simulink model "ControlFuzzy_Modelo_GA"  (R2021b)
settings: Solver=VariableStepAuto  StartTime=0.0  StopTime=300  RelTol=1e-3
values from neighbouring files (symbols this model uses):
  Kd = 0.157560742107    [optimization_Result.mat]
  Ki = 0.0257835185528    [optimization_Result.mat]
  Kp = 1.9788581039    [optimization_Result.mat]
  Ku = 1.99972376218    [optimization_Result.mat]
libraries: fuzblock x1
settings Model: Creator=diego  LastModifiedBy=diego
settings SolverCC: ZeroCrossAlgorithm=Adaptive  AlgebraicLoopSolver=TrustRegion
settings DataIOCC: SaveOutput=off  SaveTime=off  ReturnWorkspaceOutputs=off
settings DebuggingCC: IgnoredZcDiagnostic=none  SFMachineParentedDataDiag=warning

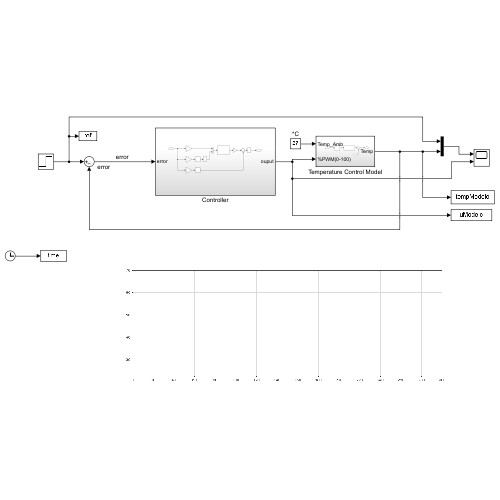
[thumbnail: Simulink's stored preview of the top-level diagram]
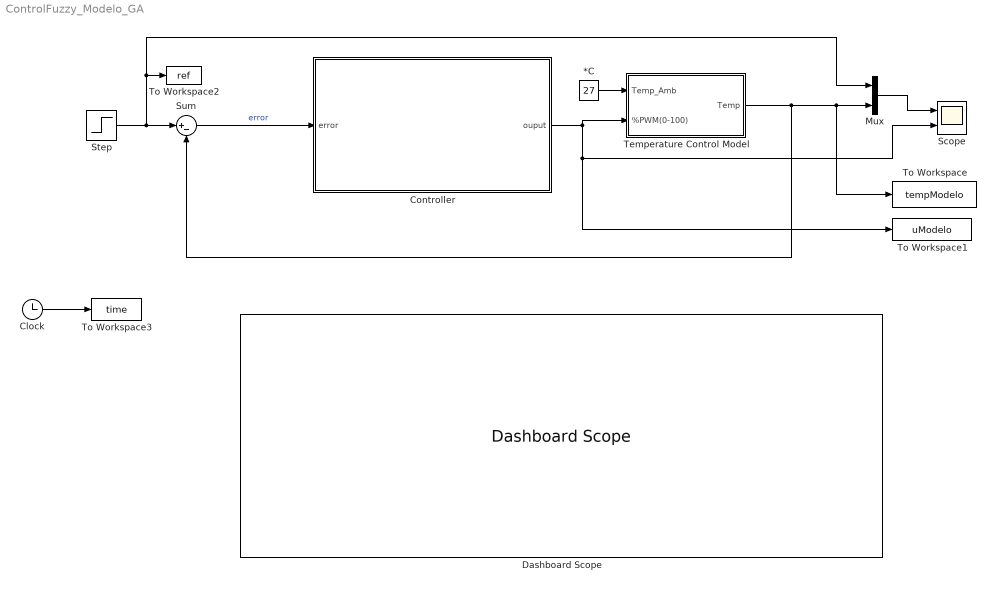
== system ControlFuzzy_Modelo_GA ==
  *C : Constant  Value=27
  Clock : Clock
  Controller : Subsystem
  Dashboard Scope : DashboardScope  Ymin=23  Ymax=70  ScaleAtStop=off
  Mux : Mux  Inputs=2
  Scope : Scope  NumInputPorts=2
  Step : Step  Before=27  After=55  SampleTime=0
  Sum : Sum  Inputs=|+-
  Temperature Control Model : Subsystem
  To Workspace : ToWorkspace  VariableName=tempModelo  SampleTime=1
      settings: Save2DSignal=2-D array (concatenate along first dimension)
  To Workspace1 : ToWorkspace  VariableName=uModelo  SampleTime=1
      settings: Save2DSignal=2-D array (concatenate along first dimension)
  To Workspace2 : ToWorkspace  VariableName=ref  SampleTime=1
      settings: Save2DSignal=2-D array (concatenate along first dimension)
  To Workspace3 : ToWorkspace  VariableName=time  SampleTime=1
      settings: Save2DSignal=2-D array (concatenate along first dimension)
  wires:
  *C/1 -> Temperature Control Model/1(Temp_Amb)
  Temperature Control Model/1(Temp) -> Sum/2, Mux/2, To Workspace/1
  Mux/1 -> Scope/1
  Step/1 -> Mux/1, To Workspace2/1, Sum/1
  Clock/1 -> To Workspace3/1
  Controller/1(ouput) -> Temperature Control Model/2(%PWM(0-100)), Scope/2, To Workspace1/1
  Sum/1 -> Controller/1(error)  "error"

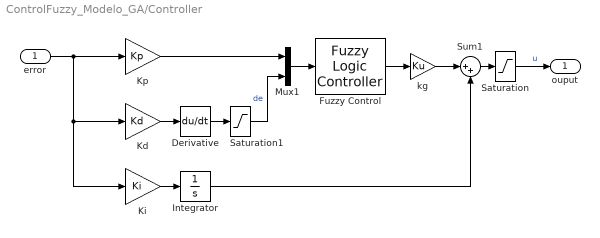
== system ControlFuzzy_Modelo_GA/Controller ==
  error : Inport
  Derivative : Derivative
  Fuzzy Control : fuzblock/Fuzzy Logic  Controller  FIS='C_Fuzzy_u100.fis'  OutputSampleNumber=101  DataType=double  FuzzifiedInputs=off  RuleFiringStrengths=off  RuleOutputs=off  AggregatedOutputs=off  SimulateUsing=Interpreted execution  OutOfRangeInputValueMessage=warning  NoRuleFiredMessage=warning  EmptyOutputFuzzySetMessage=warning
  Integrator : Integrator
  Kd : Gain  Gain=Kd
  Ki : Gain  Gain=Ki
  Kp : Gain  Gain=Kp
  Mux1 : Mux  Inputs=2
  Saturation : Saturate  UpperLimit=100  LowerLimit=0
  Saturation1 : Saturate  UpperLimit=6  LowerLimit=-6
  Sum1 : Sum  Inputs=|++
  kg : Gain  Gain=Ku
  ouput : Outport
  wires:
  Derivative/1 -> Saturation1/1
  kg/1 -> Sum1/1
  Mux1/1 -> Fuzzy Control/1
  Kd/1 -> Derivative/1
  Kp/1 -> Mux1/1
  Fuzzy Control/1 -> kg/1
  Ki/1 -> Integrator/1
  error/1 -> Kd/1, Ki/1, Kp/1
  Saturation1/1 -> Mux1/2  "de"
  Integrator/1 -> Sum1/2
  Sum1/1 -> Saturation/1
  Saturation/1 -> ouput/1  "u"

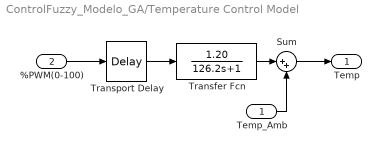
== system ControlFuzzy_Modelo_GA/Temperature Control Model ==
  Temp_Amb : Inport
  %PWM(0-100) : Inport  Port=2
  Sum : Sum  Inputs=|++
  Transfer Fcn : TransferFcn  Numerator=[1.20]  Denominator=[126.2, 1]
  Transport Delay : TransportDelay  DelayTime=14.23
  Temp : Outport
  wires:
  Transport Delay/1 -> Transfer Fcn/1
  Temp_Amb/1 -> Sum/2
  Sum/1 -> Temp/1
  Transfer Fcn/1 -> Sum/1
  %PWM(0-100)/1 -> Transport Delay/1
